simulink library "SUB_ECU_L4_MABX_HW_Interface_PIC_PB"  (R2018a)
settings: Solver=VariableStepAuto  StartTime=0.0  StopTime=10.0  RelTol=1e-3
PostLoadFcn:
  | , if any(exist('dsrtsu_mdlpostloadfcn', 'file') == [2, 3, 6]), try dsrtsu_mdlpostloadfcn('Execute', bdroot); catch fprintf('Error in PostLoadFcn (dsrtsu_mdlpostloadfcn) for model "%s":\n %s\n', bdroot, lasterr); end, end,
undefined symbols (not defined in the file or in its folder): CANR_PROPB_REAX_3_13_CHANNEL_APV, CANR_PROPB_REAX_4_13_CHANNEL_APV, CANR_PROPB_XPR_1_50_CHANNEL_APV, ENUM_CAN_RX_T, ENUM_CAN_TX_T, ENUM_REAX_OPERATION_MODE_T, ENUM_SIGNAL_HEALTH_T, ENUM_XBR_CONTROL_MODE_T, ENUM_XBR_EBI_MODE_T, ENUM_XBR_PASS_THROUGH_ACTIVE_T, ENUM_XBR_PRIORITY_T, ENUM_XPR_INHIBIT_PARK_MANUAL_T, ENUM_XPR_INHIBIT_UNPARK_MANUAL_T, ENUM_XPR_PARK_MANUAL_T, ENUM_XPR_UNPARK_MANUAL_T, PROPB_REAX_1_E4_DES_POS_SIG_SRC_APV, PROPB_REAX_1_E4_DESIRED_OPMODE_APV, PROPB_REAX_1_E4_DESIRED_POSITION_APV, PROPB_REAX_CHANNEL_APV, ptc_matlab_lib
libraries: PTC_MBDS_LIB x293, rtican x158, simulink x61, EmE_MBD_Blockset x38, rti1401lib_dio_type4 x14, simulink_need_slupdate x7, $bdroot x5, rti1401lib_adc_type4 x3, rtmapslib x3, dsa_tcpip_lib x2, SUB_ECU_L4_MABX_HW_Interface_PTC_1571 x1, rtitasklib x1
(part 19 of 49)

== system SUB_ECU_L4_MABX_HW_Interface_PIC_PB/CAN_PIC_PB/CAN_RX_TC1_05/RX_CAN_5 ==
  Enable : Inport
  Bus Creator3 : BusCreator  Inputs=28
  Data Type Conversion10 : DataTypeConversion  OutDataTypeStr=double  SaturateOnIntegerOverflow=on
  Data Type Conversion8 : DataTypeConversion  OutDataTypeStr=boolean  SaturateOnIntegerOverflow=on
  Data Type Conversion9 : DataTypeConversion  OutDataTypeStr=double  SaturateOnIntegerOverflow=on
  TC1_03_05 : rtican/RTICAN Receive (RX)   Reserved1=[]  Reserved2=[]  Reserved3=[]  Reserved4=[]  SfcnMessage=[]  Msg_Struct=[]  BoardTypeNo=[]  BoardNo=[]  ChannelNo=[]  Parameters=[]  DialogFcn=[]  UnitName=[]  Revision=[]  UnitValues=[]  DSProperties=struct('RTI',struct('Version',uint32(5),'BlockType',struct('isSLSource',uint8(1),'isSLSink',uint8(1),'isHWSource',uint8(0),'isHWSink',uint8(0),'isSetup',uint8(0),'isInline',uint8(1),'isNonInline',uint8(0),'isInterrupt',uint8(0),'isChannelwise',uint8(0)),'IOBoardType','RTICAN','UnitType','MESSAGE','Identifier','RX','DialogType','MSVC','BlockSet','RTICAN','SlaveProcessor','CAN'))  RTIBlockInterface=struct('OutputPortsWidth',int32([1 1 1 1 1 1 1 1 1 1 1 1 1 1 1 1 1 1 1 1 1 1 1 1 1 1 1 1]),'OutputPortsActive',ones(1,28),'OutputPortsName',{{'SPN681_TransGearShiftInhibitReq','SPN682_TransTrqConvLockupDisReq','SPN683_DisengageDrivelineReq','SPN4242_TransRevGearShiftInhibRq','SPN684_RequestedPercClutchSlip','SPN525_TransRequestedGear','SPN685_DisengageDiffLockRqFrAx1','SPN686_DisengageDiffLockRqFrAx2','SPN687_DisengageDiffLockRqRrAx1','SPN688_DisengageDiffLockRqRrAx2','SPN689_DisengageDiffLockRqC','SPN690_DisengageDiffLockRqCF','SPN691_DisengageDiffLockRqCR','SPN5762_TransLoadRedInhibitRq','SPN1852_TransmissionMode1','SPN1853_TransmissionMode2','SPN1854_TransmissionMode3','SPN1855_TransmissionMode4','SPN7695_TransAutoNeutralRequest','SPN4255_TransRequestedLaunchGear','SPN2985_TransShiftSelDispModeSw','SPN4246_TransmissionMode5','SPN4247_TransmissionMode6','SPN4248_TransmissionMode7','SPN4249_TransmissionMode8',['RX status'],['RX time'],['RX delta time']}},'OutputPortsDataType',{{'SS_DOUBLE','SS_DOUBLE','SS_DOUBLE','SS_DOUBLE','SS_DOUBLE','SS_DOUBLE','SS_DOUBLE','SS_DOUBLE','SS_DOUBLE','SS_DOUBLE','SS_DOUBLE','SS_DOUBLE','SS_DOUBLE','SS_DOUBLE','SS_DOUBLE','SS_DOUBLE','SS_DOUBLE','SS_DOUBLE','SS_DOUBLE','SS_DOUBLE','SS_DOUBLE','SS_DOUBLE','SS_DOUBLE','SS_DOUBLE','SS_DOUBLE','SS_DOUBLE','SS_DOUBLE','SS_DOUBLE'}},'OutputPortsLabel',{{'SPN681_TransGearShiftInhibitReq','SPN682_TransTrqConvLockupDisReq','SPN683_DisengageDrivelineReq','SPN4242_TransRevGearShiftInhibRq','SPN684_RequestedPercClutchSlip','SPN525_TransRequestedGear','SPN685_DisengageDiffLockRqFrAx1','SPN686_DisengageDiffLockRqFrAx2','SPN687_DisengageDiffLockRqRrAx1','SPN688_DisengageDiffLockRqRrAx2','SPN689_DisengageDiffLockRqC','SPN690_DisengageDiffLockRqCF','SPN691_DisengageDiffLockRqCR','SPN5762_TransLoadRedInhibitRq','SPN1852_TransmissionMode1','SPN1853_TransmissionMode2','SPN1854_TransmissionMode3','SPN1855_TransmissionMode4','SPN7695_TransAutoNeutralRequest','SPN4255_TransRequestedLaunchGear','SPN2985_TransShiftSelDispModeSw','SPN4246_TransmissionMode5','SPN4247_TransmissionMode6','SPN4248_TransmissionMode7','SPN4249_TransmissionMode8','','',''}},'OutputPortsLabelMode','ON','InputPortsWidth',int32(0),'InputPortsActive',0,'DialogFcn','rtican_message_interface_gui','BlockDisplay',{{'','center'}},'IconTransparency','on','ParameterTunableNames',{{}},'InitLevel',3,'BlockName',struct('Token',{{'TC1_03_05'}}),'SampleTime',{{-1}},'TriggerPort',{{'none'}},'EnablePort',{{'yes'}})  RTIBlockParameters="struct('BoardTypeNo',{{1,'OFF',[]}},'BoardNo',{{3,'ON',[1 16]}},'ChannelNo',{{1,'ON',[1 2]}},'Parameters',{{struct('DataFileSupport',struct('DataFileSelectedMaster',1,'DataFileSelectedLocal',0,'DataFileName',['c:\\users\\gavin.coelho\\repos\\l4 svn\\branches\\gennaro\\project_l4\\src\\projectlibrary\\dbc\\mabx_can4_chrisbaltonallstandard.dbc|c:\\users\\gavin.coelho\\repos\\l4 svn\\branches\\gennaro\\project_l4\\src\\projectlibrary\\dbc\\mabx_can4.dbc|'],'DataFileDate',{{{''}}},'SelectedFile',['<no file selected>']),'Options',struct('StatusSelected',1,'TimeSelected',1,'DeltaTimeSelected',1,'BytePortSelected',0,'MessageLengthSelected',0,'TriggerPort',struct('Selected',0,'TriggerType',0),'UserCoding',struct('Selected',0,'InterfaceFile','UserDecodingFile','FcnName','UserDecodeFcn','InportSelected',0,'InportWidth',1,'OutportSelected',0,'OutportWidth',1),'EnablePortSelected',1,'SignalOnPortnameSelected',1,'UseRXService',1),'Message',struct('MsgOnBlocknameSelected',1,'MsgName','TC1_03_05','MsgIdFormat',1,'MsgId',201392901,'MsgLength',8,'NumSignals',25,'SampleTime',-1,'Signal',struct('SgnName',{'SPN681_TransGearShiftInhibitReq','SPN682_TransTrqConvLockupDisReq','SPN683_DisengageDrivelineReq','SPN4242_TransRevGearShiftInhibRq','SPN684_RequestedPercClutchSlip','SPN525_TransRequestedGear','SPN685_DisengageDiffLockRqFrAx1','SPN686_DisengageDiffLockRqFrAx2','SPN687_DisengageDiffLockRqRrAx1','SPN688_DisengageDiffLockRqRrAx2','SPN689_DisengageDiffLockRqC','SPN690_DisengageDiffLockRqCF','SPN691_DisengageDiffLockRqCR','SPN5762_TransLoadRedInhibitRq','SPN1852_TransmissionMode1','SPN1853_TransmissionMode2','SPN1854_TransmissionMode3','SPN1855_TransmissionMode4','SPN7695_TransAutoNeutralRequest','SPN4255_TransRequestedLaunchGear','SPN2985_TransShiftSelDispModeSw','SPN4246_TransmissionMode5','SPN4247_TransmissionMode6','SPN4248_TransmissionMode7','SPN4249_TransmissionMode8'},'SgnStartBit',{0,2,4,6,8,16,24,26,28,30,32,34,36,38,40,42,44,46,48,50,54,56,58,60,62},'SgnLength',{2,2,2,2,8,8,2,2,2,2,2,2,2,2,2,2,2,2,2,4,2,2,2,2,2},'SgnType',{0,0,0,0,0,0,0,0,0,0,0,0,0,0,0,0,0,0,0,0,0,0,0,0,0},'ModeValue',{-1,-1,-1,-1,-1,-1,-1,-1,-1,-1,-1,-1,-1,-1,-1,-1,-1,-1,-1,-1,-1,-1,-1,-1,-1},'DataType',{0,0,0,0,0,0,0,0,0,0,0,0,0,0,0,0,0,0,0,0,0,0,0,0,0},'ByteLayout',{0,0,0,0,0,0,0,0,0,0,0,0,0,0,0,0,0,0,0,0,0,0,0,0,0},'Factor',{1,1,1,1,0.4,1,1,1,1,1,1,1,1,1,1,1,1,1,1,1,1,1,1,1,1},'Offset',{0,0,0,0,0,-125,0,0,0,0,0,0,0,0,0,0,0,0,0,0,0,0,0,0,0},'SgnComment',{{['Command signal to inhibit gear shifts.']},{['Command signal to prevent torque converter lockup, which may cause problems in certain circumstances for ASR.']},{''},{['Allows devices external to the normal transmission shift selector system to request the transmission to inhibit shifts into any Reverse gear and force the transmission into Neutral if it is currently in Reverse or attempting to shift to Reverse.']},{['Parameter which represents the percent clutch slip requested by a device.']},{['Gear requested by the operator, ABS, or engine.']},{['Command signal used to disengage the various differential locks, e.g., to allow an undistributed individual wheel control by ABS.  The differential locks are located as defined in Figure SPN564_A.']},{['Command signal used to disengage the various differential locks, e.g., to allow an undistributed individual wheel control by ABS.  The differential locks are located as defined in Figure SPN564_A']},{['Command signal used to disengage the various differential locks, e.g., to allow an undistributed individual wheel control by ABS.  The differential locks are located as defined in Figure SPN564_A']},{['Command signal used to disengage the various differential locks, e.g., to allow an undistributed individual wheel control by ABS.  The differential locks are located as defined in Figure SPN564_A']},{['Command signal used to disengage the various differential locks, e.g., to allow an undistributed individual wheel control by ABS.  The differential locks are located as defined in Figure SPN564_A']},{['Command signal used to disengage the various differential locks, e.g., to allow an undistributed individual wheel control by ABS.  The differential locks are located as defined in Figure SPN564_A.']},{['Command signal used to disengage the various differential locks, e.g., to allow an undistributed individual wheel control by ABS.  The differential locks are located as defined in Figure SPN564_A.']},{['Request signal to the transmission to inhibit activation of load reduction functions.']},{['Indicates whether transmission mode 1 is enabled.  Modes are manufacturer specific and are not necessarily mutually exclusive.  See also SPN 2536.']},{['Indicates whether transmission mode 2 is enabled.  Modes are manufacturer specific and are not necessarily mutually exclusive.  See also SPN 2537.']},{['Indicates whether transmission mode 3 is enabled.  Modes are manufacturer specific and are not necessarily mutually exclusive.  See also SPN 2538.']},{['Indicates whether transmission mode 4 is enabled.  Modes are manufacturer specific and are not necessarily mutually exclusive.  See also SPN 2539.']},{['This parameter conveys a vehicle system desire to override the operator’s current shift selector request (e.g. Drive, Reverse) and shift the transmission into Neutral']},{['Initial gear for the transmission to start out in when the vehicle is launched from a standing stop, as specified by the vehicle operator or vehicle system.']},{['Status of the operator’s switch used to ‘toggle’ through multiple display modes of a shift selector display.']},{['Indicates whether transmission mode 5 is enabled. Modes are manufacturer specific and are not necessarily mutually exclusive. See also SPN 4250.']},{['Indicates whether transmission mode 6 is enabled. Modes are manufacturer specific and are not necessarily mutually exclusive. See also SPN 4251.']},{['Indicates whether transmission mode 7 is enabled. Modes are manufacturer specific and are not necessarily mutually exclusive. See also SPN 4252.']},{['Indicates whether transmission mode 8 is enabled. Modes are manufacturer specific and are not necessarily mutually exclusive. See also SPN 4253.']}},'SgnUnit',{'','','','','%','','','','','','','','','','','','','','','','','','','',''},'Min',{0,0,0,0,0,0,0,0,0,0,0,0,0,0,0,0,0,0,0,0,0,0,0,0,0},'Max',{0,0,0,0,0,0,0,0,0,0,0,0,0,0,0,0,0,0,0,0,0,0,0,0,0},'SLDataType',{'SS_DOUBLE','SS_DOUBLE','SS_DOUBLE','SS_DOUBLE','SS_DOUBLE','SS_DOUBLE','SS_DOUBLE','SS_DOUBLE','SS_DOUBLE','SS_DOUBLE','SS_DOUBLE','SS_DOUBLE','SS_DOUBLE','SS_DOUBLE','SS_DOUBLE','SS_DOUBLE','SS_DOUBLE','SS_DOUBLE','SS_DOUBLE','SS_DOUBLE','SS_DOUBLE','SS_DOUBLE','SS_DOUBLE','SS_DOUBLE','SS_DOUBLE'}),'MsgIdNumFormat',1,'MsgComment',{{['Transmission Control 1']}}),'Version',1.2,'general',struct('isFromLib',0)),'OFF',[]}},'GroupId',{{struct('Group',{{'RTICAN'}},'No',5,'Behavior',{{'NAMECHANGE'}},'BlockType',{{'SINK'}},'NameChangeFlag',0),'OFF',[]}},'SFcnRTICANMessage',{{struct('MsgType','RX','SFcnPortType','Scalar','MsgName','TC1_03_05','MsgIdFormat','XTD','MsgId',201392901,'MsgLength',8,'NumSignals',25,'SampleTime',-1,'Signal',struct('SgnName',{'SPN681_TransGearShiftInhibitReq','SPN682_TransTrqConvLockupDisReq','SPN683_DisengageDrivelineReq','SPN4242_TransRevGearShiftInhibRq','SPN684_RequestedPercClutchSlip','SPN525_TransRequestedGear','SPN685_DisengageDiffLockRqFrAx1','SPN686_DisengageDiffLockRqFrAx2','SPN687_DisengageDiffLockRqRrAx1','SPN688_DisengageDiffLockRqRrAx2','SPN689_DisengageDiffLockRqC','SPN690_DisengageDiffLockRqCF','SPN691_DisengageDiffLockRqCR','SPN5762_TransLoadRedInhibitRq','SPN1852_TransmissionMode1','SPN1853_TransmissionMode2','SPN1854_TransmissionMode3','SPN1855_TransmissionMode4','SPN7695_TransAutoNeutralRequest','SPN4255_TransRequestedLaunchGear','SPN2985_TransShiftSelDispModeSw','SPN4246_TransmissionMode5','SPN4247_TransmissionMode6','SPN4248_TransmissionMode7','SPN4249_TransmissionMode8'},'SgnStartBit',{0,2,4,6,8,16,24,26,28,30,32,34,36,38,40,42,44,46,48,50,54,56,58,60,62},'SgnLength',{2,2,2,2,8,8,2,2,2,2,2,2,2,2,2,2,2,2,2,4,2,2,2,2,2},'SgnType',{'standard','standard','standard','standard','standard','standard','standard','standard','standard','standard','standard','standard','standard','standard','standard','standard','standard','standard','standard','standard','standard','standard','standard','standard','standard'},'ModeValue',{-1,-1,-1,-1,-1,-1,-1,-1,-1,-1,-1,-1,-1,-1,-1,-1,-1,-1,-1,-1,-1,-1,-1,-1,-1},'DataType',{['unsigned int'],['unsigned int'],['unsigned int'],['unsigned int'],['unsigned int'],['unsigned int'],['unsigned int'],['unsigned int'],['unsigned int'],['unsigned int'],['unsigned int'],['unsigned int'],['unsigned int'],['unsigned int'],['unsigned int'],['unsigned int'],['unsigned int'],['unsigned int'],['unsigned int'],['unsigned int'],['unsigned int'],['unsigned int'],['unsigned int'],['unsigned int'],['unsigned int']},'ByteLayout',{['little endian'],['little endian'],['little endian'],['little endian'],['little endian'],['little endian'],['little endian'],['little endian'],['little endian'],['little endian'],['little endian'],['little endian'],['little endian'],['little endian'],['little endian'],['little endian'],['little endian'],['little endian'],['little endian'],['little endian'],['little endian'],['little endian'],['little endian'],['little endian'],['little endian']},'Factor',{1,1,1,1,0.4,1,1,1,1,1,1,1,1,1,1,1,1,1,1,1,1,1,1,1,1},'Offset',{0,0,0,0,0,-125,0,0,0,0,0,0,0,0,0,0,0,0,0,0,0,0,0,0,0},'SLDataType',{'SS_DOUBLE','SS_DOUBLE','SS_DOUBLE','SS_DOUBLE','SS_DOUBLE','SS_DOUBLE','SS_DOUBLE','SS_DOUBLE','SS_DOUBLE','SS_DOUBLE','SS_DOUBLE','SS_DOUBLE','SS_DOUBLE','SS_DOUBLE','SS_DOUBLE','SS_DOUBLE','SS_DOUBLE','SS_DOUBLE','SS_DOUBLE','SS_DOUBLE','SS_DOUBLE','SS_DOUBLE','SS_DOUBLE','SS_DOUBLE','SS_DOUBLE'}),'StatusSelected','yes','TimeSelected','yes','DeltaTimeSelected','yes','BytePortSelected','no','MessageLengthSelected','no','TriggerPort',struct('Selected','no','TriggerType',0),'UserCoding',struct('Selected','no','InterfaceFile','UserDecodingFile','FcnName','UserDecodeFcn','InportSelected','no','InportWidth',1,'OutportSelected','no','OutportWidth',1),'EnablePortSelected','yes','UseRXService','yes','BoardType','DS1','BoardNo',3,'ControllerNo',1),'OFF',[]}},'TLCFileName',{{'rtican_rx_message','OFF',[]}})"  RTISFcnParameters=struct('SFcnRTICANMessage','struct','TLCFileName','char')  RTIBlockParaDefault=struct('BoardTypeNo',4302,'BoardNo',1,'ChannelNo',1,'Parameters',struct('DataFileSupport',struct('DataFileSelectedMaster',0,'DataFileSelectedLocal',0,'DataFileName','','DataFileDate','','SelectedFile',['<no file selected>']),'Options',struct('StatusSelected',1,'TimeSelected',1,'DeltaTimeSelected',1,'BytePortSelected',0,'MessageLengthSelected',0,'TriggerPort',struct('Selected',0,'TriggerType','rising'),'UserCoding',struct('Selected',0,'InterfaceFile','UserDecodingFile','FcnName','UserDecodeFcn','InportSelected',0,'InportWidth',1,'OutportSelected',0,'OutportWidth',1),'EnablePortSelected',0,'SignalOnPortnameSelected',1,'UseRXService',0),'Message',struct('MsgOnBlocknameSelected',0,'MsgName',['RX Message'],'MsgIdFormat',0,'MsgId',100,'MsgLength',8,'NumSignals',1,'SampleTime',-1,'Signal',struct('SgnName',['RX signal'],'SgnStartBit',0,'SgnLength',8,'SgnType',0,'ModeValue',-1,'DataType',0,'SLDataType','SS_DOUBLE','ByteLayout',0,'Factor',1,'Offset',0,'Min',0,'Max',255,'SgnComment',{{}},'SgnUnit',''),'MsgIdNumFormat',0,'MsgComment',{{''}}),'Version',1.2,'general',struct('isFromLib',1)),'GroupId',struct('Group',{{'RTICAN'}},'No',1,'Behavior',{{'NAMECHANGE'}},'BlockType',{{'SINK'}},'NameChangeFlag',0),'SFcnRTICANMessage',struct('MsgType','RX','MsgName',['RX Message'],'MsgIdFormat','STD','MsgId',100,'MsgLength',8,'NumSignals',1,'SampleTime',-1,'Signal',struct('SgnName',['RX signal'],'SgnStartBit',0,'SgnLength',8,'SgnType','standard','ModeValue',-1,'DataType',['unsigned int'],'ByteLayout',['little endian'],'SLDataType','SS_DOUBLE','Factor',1,'Offset',0),'StatusSelected','yes','TimeSelected','yes','DeltaTimeSelected','yes','BytePortSelected','no','MessageLengthSelected','no','EnablePortSelected','no','UserCoding',struct('Selected','no','InterfaceFile','UserDecodingFile','FcnName','UserDecodeFcn','InportSelected','no','InportWidth',1,'OutportSelected','no','OutportWidth',1),'TriggerPort',struct('Selected','no','TriggerType','rising'),'UseRXService','no','BoardType','DS4302','BoardNo',1,'ControllerNo',1,'SFcnPortType','Scalar'),'TLCFileName','rtican_rx_message')
      settings: AttributesFormatString=Group Id: RTICAN5\n  SourceProductName=dSPACE RTI CAN Blockset
  TC1_05 : Outport
  wires:
  Data Type Conversion9/1 -> Bus Creator3/27  "RX_time"
  Data Type Conversion10/1 -> Bus Creator3/28  "RX_delta_time"
  Data Type Conversion8/1 -> Bus Creator3/26  "RX_status"
  TC1_03_05/26 -> Data Type Conversion8/1
  TC1_03_05/27 -> Data Type Conversion9/1
  TC1_03_05/28 -> Data Type Conversion10/1
  Enable/1 -> TC1_03_05/Enable
  Bus Creator3/1 -> TC1_05/1  "TC1_05"
  TC1_03_05/23 -> Bus Creator3/23  "SPN4247_TransmissionMode6"
  TC1_03_05/24 -> Bus Creator3/24  "SPN4248_TransmissionMode7"
  TC1_03_05/25 -> Bus Creator3/25  "SPN4249_TransmissionMode8"
  TC1_03_05/22 -> Bus Creator3/22  "SPN4246_TransmissionMode5"
  TC1_03_05/21 -> Bus Creator3/21  "SPN2985_TransShiftSelDispModeSw"
  TC1_03_05/7 -> Bus Creator3/7  "SPN685_DisengageDiffLockRqFrAx1"
  TC1_03_05/18 -> Bus Creator3/18  "SPN1855_TransmissionMode4"
  TC1_03_05/19 -> Bus Creator3/19  "SPN7695_TransAutoNeutralRequest"
  TC1_03_05/8 -> Bus Creator3/8  "SPN686_DisengageDiffLockRqFrAx2"
  TC1_03_05/12 -> Bus Creator3/12  "SPN690_DisengageDiffLockRqCF"
  TC1_03_05/16 -> Bus Creator3/16  "SPN1853_TransmissionMode2"
  TC1_03_05/9 -> Bus Creator3/9  "SPN687_DisengageDiffLockRqRrAx1"
  TC1_03_05/10 -> Bus Creator3/10  "SPN688_DisengageDiffLockRqRrAx2"
  TC1_03_05/11 -> Bus Creator3/11  "SPN689_DisengageDiffLockRqC"
  TC1_03_05/13 -> Bus Creator3/13  "SPN691_DisengageDiffLockRqCR"
  TC1_03_05/20 -> Bus Creator3/20  "SPN4255_TransRequestedLaunchGear"
  TC1_03_05/15 -> Bus Creator3/15  "SPN1852_TransmissionMode1"
  TC1_03_05/17 -> Bus Creator3/17  "SPN1854_TransmissionMode3"
  TC1_03_05/14 -> Bus Creator3/14  "SPN5762_TransLoadRedInhibitRq"
  TC1_03_05/3 -> Bus Creator3/3  "SPN683_DisengageDrivelineReq"
  TC1_03_05/6 -> Bus Creator3/6  "SPN525_TransRequestedGear"
  TC1_03_05/4 -> Bus Creator3/4  "SPN4242_TransRevGearShiftInhibRq"
  TC1_03_05/5 -> Bus Creator3/5  "SPN684_RequestedPercClutchSlip"
  TC1_03_05/1 -> Bus Creator3/1  "SPN681_TransGearShiftInhibitReq"
  TC1_03_05/2 -> Bus Creator3/2  "SPN682_TransTrqConvLockupDisReq"

== system SUB_ECU_L4_MABX_HW_Interface_PIC_PB/CAN_PIC_PB/CAN_RX_VDC1_0B/RX_CAN_1 ==
  Enable : Inport
  Bus Creator3 : BusCreator  Inputs=10
  Data Type Conversion10 : DataTypeConversion  OutDataTypeStr=double  SaturateOnIntegerOverflow=on
  Data Type Conversion8 : DataTypeConversion  OutDataTypeStr=boolean  SaturateOnIntegerOverflow=on
  Data Type Conversion9 : DataTypeConversion  OutDataTypeStr=double  SaturateOnIntegerOverflow=on
  VDC1_0B_ : rtican/RTICAN Receive (RX)   Reserved1=[]  Reserved2=[]  Reserved3=[]  Reserved4=[]  SfcnMessage=[]  Msg_Struct=[]  BoardTypeNo=[]  BoardNo=[]  ChannelNo=[]  Parameters=[]  DialogFcn=[]  UnitName=[]  Revision=[]  UnitValues=[]  DSProperties=struct('RTI',struct('Version',uint32(5),'BlockType',struct('isSLSource',uint8(1),'isSLSink',uint8(1),'isHWSource',uint8(0),'isHWSink',uint8(0),'isSetup',uint8(0),'isInline',uint8(1),'isNonInline',uint8(0),'isInterrupt',uint8(0),'isChannelwise',uint8(0)),'IOBoardType','RTICAN','UnitType','MESSAGE','Identifier','RX','DialogType','MSVC','BlockSet','RTICAN','SlaveProcessor','CAN'))  RTIBlockInterface=struct('OutputPortsWidth',int32([1 1 1 1 1 1 1 1 1 1]),'OutputPortsActive',[1 1 1 1 1 1 1 1 1 1],'OutputPortsName',{{'VDCInformationSignal','VDCFullyOperational','VDCBrakeLightRq','ROPEngCtrlActive','ROPBrakeCtrlActive','YCEngCtrlActive','YCBrakeCtrlActive',['RX status'],['RX time'],['RX delta time']}},'OutputPortsDataType',{{'SS_DOUBLE','SS_DOUBLE','SS_DOUBLE','SS_DOUBLE','SS_DOUBLE','SS_DOUBLE','SS_DOUBLE','SS_DOUBLE','SS_DOUBLE','SS_DOUBLE'}},'OutputPortsLabel',{{'VDCInformationSignal','VDCFullyOperational','VDCBrakeLightRq','ROPEngCtrlActive','ROPBrakeCtrlActive','YCEngCtrlActive','YCBrakeCtrlActive','','',''}},'OutputPortsLabelMode','ON','InputPortsWidth',int32(0),'InputPortsActive',0,'DialogFcn','rtican_message_interface_gui','BlockDisplay',{{'','center'}},'IconTransparency','on','ParameterTunableNames',{{}},'InitLevel',3,'BlockName',struct('Token',{{'VDC1_0B'}}),'SampleTime',{{-1}},'TriggerPort',{{'none'}},'EnablePort',{{'yes'}})  RTIBlockParameters=struct('BoardTypeNo',{{1,'OFF',[]}},'BoardNo',{{1,'ON',[1 16]}},'ChannelNo',{{1,'ON',[1 2]}},'Parameters',{{struct('DataFileSupport',struct('DataFileSelectedMaster',1,'DataFileSelectedLocal',0,'DataFileName',['c:\users\gavin.coelho\repos\l4 svn\branches\gennaro\project_l4\src\projectlibrary\dbc\mabx_can1.dbc|c:\users\gavin.coelho\repos\l4 svn\branches\gennaro\project_l4\src\projectlibrary\dbc\j1939_famosdbcwithfusion.dbc|'],'DataFileDate',{{{['31-Jan-2018 07:14:07']},{['31-Jan-2018 07:14:07']}}},'SelectedFile','dbc\j1939_famosdbcwithfusion.dbc','InterfaceFcn','rtican_dbc_file_parser'),'Options',struct('StatusSelected',1,'TimeSelected',1,'DeltaTimeSelected',1,'BytePortSelected',0,'MessageLengthSelected',0,'TriggerPort',struct('Selected',0,'TriggerType',0),'UserCoding',struct('Selected',0,'InterfaceFile','UserDecodingFile','FcnName','UserDecodeFcn','InportSelected',0,'InportWidth',1,'OutportSelected',0,'OutportWidth',1),'EnablePortSelected',1,'SignalOnPortnameSelected',1,'UseRXService',1),'Message',struct('MsgOnBlocknameSelected',1,'MsgName','VDC1_0B','MsgIdFormat',1,'MsgId',419319563,'MsgLength',8,'NumSignals',7,'SampleTime',-1,'Signal',struct('SgnName',{'VDCInformationSignal','VDCFullyOperational','VDCBrakeLightRq','ROPEngCtrlActive','ROPBrakeCtrlActive','YCEngCtrlActive','YCBrakeCtrlActive'},'SgnStartBit',{0,2,4,8,10,12,14},'SgnLength',{2,2,2,2,2,2,2},'SgnType',{0,0,0,0,0,0,0},'ModeValue',{-1,-1,-1,-1,-1,-1,-1},'DataType',{0,0,0,0,0,0,0},'ByteLayout',{0,0,0,0,0,0,0},'Factor',{1,1,1,1,1,1,1},'Offset',{0,0,0,0,0,0,0},'SgnComment',{{['This parameter commands the VDC information signal, for example a dash lamp.']},{['Signal that indicates whether VDC is fully operational or whether its functionality is reduced by a permanent or temporary']},{['Indicates whether VDC requests to turn the vehicle brake lights on']},{['State Signal which indicates that the Roll Over Prevention (ROP) has commanded engine control to be active.']},{['State signal which indicates that Roll over Prevention (ROP) has activated brake control.']},{['State Signal which indicates that the Yaw Control (YC) has commanded engine control to be active.']},{['State signal which indicates that Yaw Control (YC) has activated brake control.']}},'SgnUnit',{'','','','','','',''},'Min',{0,0,0,0,0,0,0},'Max',{3,3,3,3,3,3,3},'SLDataType',{'SS_DOUBLE','SS_DOUBLE','SS_DOUBLE','SS_DOUBLE','SS_DOUBLE','SS_DOUBLE','SS_DOUBLE'}),'MsgIdNumFormat',1,'MsgComment',{{['Vehicle Dynamic Stability Control 1']}}),'Version',1.2,'general',struct('isFromLib',0)),'OFF',[]}},'GroupId',{{struct('Group',{{'RTICAN'}},'No',1,'Behavior',{{'NAMECHANGE'}},'BlockType',{{'SINK'}},'NameChangeFlag',0),'OFF',[]}},'SFcnRTICANMessage',{{struct('MsgType','RX','SFcnPortType','Scalar','MsgName','VDC1_0B','MsgIdFormat','XTD','MsgId',419319563,'MsgLength',8,'NumSignals',7,'SampleTime',-1,'Signal',struct('SgnName',{'VDCInformationSignal','VDCFullyOperational','VDCBrakeLightRq','ROPEngCtrlActive','ROPBrakeCtrlActive','YCEngCtrlActive','YCBrakeCtrlActive'},'SgnStartBit',{0,2,4,8,10,12,14},'SgnLength',{2,2,2,2,2,2,2},'SgnType',{'standard','standard','standard','standard','standard','standard','standard'},'ModeValue',{-1,-1,-1,-1,-1,-1,-1},'DataType',{['unsigned int'],['unsigned int'],['unsigned int'],['unsigned int'],['unsigned int'],['unsigned int'],['unsigned int']},'ByteLayout',{['little endian'],['little endian'],['little endian'],['little endian'],['little endian'],['little endian'],['little endian']},'Factor',{1,1,1,1,1,1,1},'Offset',{0,0,0,0,0,0,0},'SLDataType',{'SS_DOUBLE','SS_DOUBLE','SS_DOUBLE','SS_DOUBLE','SS_DOUBLE','SS_DOUBLE','SS_DOUBLE'}),'StatusSelected','yes','TimeSelected','yes','DeltaTimeSelected','yes','BytePortSelected','no','MessageLengthSelected','no','TriggerPort',struct('Selected','no','TriggerType',0),'UserCoding',struct('Selected','no','InterfaceFile','UserDecodingFile','FcnName','UserDecodeFcn','InportSelected','no','InportWidth',1,'OutportSelected','no','OutportWidth',1),'EnablePortSelected','yes','UseRXService','yes','BoardType','DS1','BoardNo',1,'ControllerNo',1),'OFF',[]}},'TLCFileName',{{'rtican_rx_message','OFF',[]}})  RTISFcnParameters=struct('SFcnRTICANMessage','struct','TLCFileName','char')  RTIBlockParaDefault=struct('BoardTypeNo',4302,'BoardNo',1,'ChannelNo',1,'Parameters',struct('DataFileSupport',struct('DataFileSelectedMaster',0,'DataFileSelectedLocal',0,'DataFileName','','DataFileDate','','SelectedFile',['<no file selected>']),'Options',struct('StatusSelected',1,'TimeSelected',1,'DeltaTimeSelected',1,'BytePortSelected',0,'MessageLengthSelected',0,'TriggerPort',struct('Selected',0,'TriggerType','rising'),'UserCoding',struct('Selected',0,'InterfaceFile','UserDecodingFile','FcnName','UserDecodeFcn','InportSelected',0,'InportWidth',1,'OutportSelected',0,'OutportWidth',1),'EnablePortSelected',0,'SignalOnPortnameSelected',1,'UseRXService',0),'Message',struct('MsgOnBlocknameSelected',0,'MsgName',['RX Message'],'MsgIdFormat',0,'MsgId',100,'MsgLength',8,'NumSignals',1,'SampleTime',-1,'Signal',struct('SgnName',['RX signal'],'SgnStartBit',0,'SgnLength',8,'SgnType',0,'ModeValue',-1,'DataType',0,'SLDataType','SS_DOUBLE','ByteLayout',0,'Factor',1,'Offset',0,'Min',0,'Max',255,'SgnComment',{{}},'SgnUnit',''),'MsgIdNumFormat',0,'MsgComment',{{''}}),'Version',1.2,'general',struct('isFromLib',1)),'GroupId',struct('Group',{{'RTICAN'}},'No',1,'Behavior',{{'NAMECHANGE'}},'BlockType',{{'SINK'}},'NameChangeFlag',0),'SFcnRTICANMessage',struct('MsgType','RX','MsgName',['RX Message'],'MsgIdFormat','STD','MsgId',100,'MsgLength',8,'NumSignals',1,'SampleTime',-1,'Signal',struct('SgnName',['RX signal'],'SgnStartBit',0,'SgnLength',8,'SgnType','standard','ModeValue',-1,'DataType',['unsigned int'],'ByteLayout',['little endian'],'SLDataType','SS_DOUBLE','Factor',1,'Offset',0),'StatusSelected','yes','TimeSelected','yes','DeltaTimeSelected','yes','BytePortSelected','no','MessageLengthSelected','no','EnablePortSelected','no','UserCoding',struct('Selected','no','InterfaceFile','UserDecodingFile','FcnName','UserDecodeFcn','InportSelected','no','InportWidth',1,'OutportSelected','no','OutportWidth',1),'TriggerPort',struct('Selected','no','TriggerType','rising'),'UseRXService','no','BoardType','DS4302','BoardNo',1,'ControllerNo',1,'SFcnPortType','Scalar'),'TLCFileName','rtican_rx_message')
      settings: AttributesFormatString=Group Id: RTICAN1\n  SourceProductName=dSPACE RTI CAN Blockset
  VDC1_0B : Outport
  wires:
  Data Type Conversion9/1 -> Bus Creator3/9  "RX_time"
  Data Type Conversion10/1 -> Bus Creator3/10  "RX_delta_time"
  Data Type Conversion8/1 -> Bus Creator3/8  "RX_status"
  VDC1_0B_/8 -> Data Type Conversion8/1
  VDC1_0B_/9 -> Data Type Conversion9/1
  VDC1_0B_/10 -> Data Type Conversion10/1
  Enable/1 -> VDC1_0B_/Enable
  Bus Creator3/1 -> VDC1_0B/1  "VDC1_0B"
  VDC1_0B_/1 -> Bus Creator3/1  "VDCInformationSignal"
  VDC1_0B_/2 -> Bus Creator3/2  "VDCFullyOperational"
  VDC1_0B_/3 -> Bus Creator3/3  "VDCBrakeLightRq"
  VDC1_0B_/4 -> Bus Creator3/4  "ROPEngCtrlActive"
  VDC1_0B_/5 -> Bus Creator3/5  "ROPBrakeCtrlActive"
  VDC1_0B_/6 -> Bus Creator3/6  "YCEngCtrlActive"
  VDC1_0B_/7 -> Bus Creator3/7  "YCBrakeCtrlActive"

== system SUB_ECU_L4_MABX_HW_Interface_PIC_PB/CAN_PIC_PB/CAN_RX_VDC2_0B/RX_CAN_1 ==
  Enable : Inport
  Bus Creator3 : BusCreator  Inputs=9
  Data Type Conversion10 : DataTypeConversion  OutDataTypeStr=double  SaturateOnIntegerOverflow=on
  Data Type Conversion8 : DataTypeConversion  OutDataTypeStr=boolean  SaturateOnIntegerOverflow=on
  Data Type Conversion9 : DataTypeConversion  OutDataTypeStr=double  SaturateOnIntegerOverflow=on
  VDC2_0B1 : rtican/RTICAN Receive (RX)   Reserved1=[]  Reserved2=[]  Reserved3=[]  Reserved4=[]  SfcnMessage=[]  Msg_Struct=[]  BoardTypeNo=[]  BoardNo=[]  ChannelNo=[]  Parameters=[]  DialogFcn=[]  UnitName=[]  Revision=[]  UnitValues=[]  DSProperties=struct('RTI',struct('Version',uint32(5),'BlockType',struct('isSLSource',uint8(1),'isSLSink',uint8(1),'isHWSource',uint8(0),'isHWSink',uint8(0),'isSetup',uint8(0),'isInline',uint8(1),'isNonInline',uint8(0),'isInterrupt',uint8(0),'isChannelwise',uint8(0)),'IOBoardType','RTICAN','UnitType','MESSAGE','Identifier','RX','DialogType','MSVC','BlockSet','RTICAN','SlaveProcessor','CAN'))  RTIBlockInterface=struct('OutputPortsWidth',int32([1 1 1 1 1 1 1 1 1]),'OutputPortsActive',[1 1 1 1 1 1 1 1 1],'OutputPortsName',{{'SteerWheelAngle','SteerWheelTurnCounter','SteerWheelAngleSensorType','YawRate','LateralAcceleration','LongitudinalAcceleration',['RX status'],['RX time'],['RX delta time']}},'OutputPortsDataType',{{'SS_DOUBLE','SS_DOUBLE','SS_DOUBLE','SS_DOUBLE','SS_DOUBLE','SS_DOUBLE','SS_DOUBLE','SS_DOUBLE','SS_DOUBLE'}},'OutputPortsLabel',{{'SteerWheelAngle','SteerWheelTurnCounter','SteerWheelAngleSensorType','YawRate','LateralAcceleration','LongitudinalAcceleration','','',''}},'OutputPortsLabelMode','ON','InputPortsWidth',int32(0),'InputPortsActive',0,'DialogFcn','rtican_message_interface_gui','BlockDisplay',{{'','center'}},'IconTransparency','on','ParameterTunableNames',{{}},'InitLevel',3,'BlockName',struct('Token',{{'VDC2_0B'}}),'SampleTime',{{-1}},'TriggerPort',{{'none'}},'EnablePort',{{'yes'}})  RTIBlockParameters=struct('BoardTypeNo',{{1,'OFF',[]}},'BoardNo',{{1,'ON',[1 16]}},'ChannelNo',{{1,'ON',[1 2]}},'Parameters',{{struct('DataFileSupport',struct('DataFileSelectedMaster',1,'DataFileSelectedLocal',0,'DataFileName',['c:\users\gavin.coelho\repos\l4 svn\branches\gennaro\project_l4\src\projectlibrary\dbc\mabx_can1.dbc|c:\users\gavin.coelho\repos\l4 svn\branches\gennaro\project_l4\src\projectlibrary\dbc\j1939_famosdbcwithfusion.dbc|'],'DataFileDate',['03-Apr-2017 12:55:40'],'SelectedFile',['<no file selected>'],'InterfaceFcn','rtican_dbc_file_parser'),'Options',struct('StatusSelected',1,'TimeSelected',1,'DeltaTimeSelected',1,'BytePortSelected',0,'MessageLengthSelected',0,'TriggerPort',struct('Selected',0,'TriggerType',0),'UserCoding',struct('Selected',0,'InterfaceFile','UserDecodingFile','FcnName','UserDecodeFcn','InportSelected',0,'InportWidth',1,'OutportSelected',0,'OutportWidth',1),'EnablePortSelected',1,'SignalOnPortnameSelected',1,'UseRXService',1),'Message',struct('MsgOnBlocknameSelected',1,'MsgName','VDC2_0B','MsgIdFormat',1,'MsgId',418384139,'MsgLength',8,'NumSignals',6,'SampleTime',-1,'Signal',struct('SgnName',{'SteerWheelAngle','SteerWheelTurnCounter','SteerWheelAngleSensorType','YawRate','LateralAcceleration','LongitudinalAcceleration'},'SgnStartBit',{0,16,22,24,40,56},'SgnLength',{16,6,2,16,16,8},'SgnType',{0,0,0,0,0,0},'ModeValue',{-1,-1,-1,-1,-1,-1},'DataType',{0,0,0,0,0,0},'ByteLayout',{0,0,0,0,0,0},'Factor',{2^-10,1,1,2^-13,2^-11,0.1},'Offset',{-31.374,-32,0,-3.92,-15.687,-12.5},'SgnComment',{{['The main operator`s steering wheel angle (on the steering column, not the actual wheel angle).']},{['Indicates number of steering wheel turns, absolute position or relative position at ignition on.']},{['Indicates whether the steering wheel angle sensor is capable of absolute measuring of the number of steering wheel']},{['Indicates the rotation about the vertical axis.']},{['Indicates a lateral acceleration of the vehicle.']},{['Indicates the longitudinal acceleration of the vehicle.']}},'SgnUnit',{'rad','turns','','rad/s','m/s²','m/s²'},'Min',{-31.374,-32,0,-3.92,-15.687,-12.5},'Max',{31.374,29,3,3.92,15.687,12.5},'SLDataType',{'SS_DOUBLE','SS_DOUBLE','SS_DOUBLE','SS_DOUBLE','SS_DOUBLE','SS_DOUBLE'}),'MsgIdNumFormat',1,'MsgComment',{{['Vehicle Dynamic Stability Control 2']}}),'Version',1.2,'general',struct('isFromLib',0)),'OFF',[]}},'GroupId',{{struct('Group',{{'RTICAN'}},'No',1,'Behavior',{{'NAMECHANGE'}},'BlockType',{{'SINK'}},'NameChangeFlag',0),'OFF',[]}},'SFcnRTICANMessage',{{struct('MsgType','RX','SFcnPortType','Scalar','MsgName','VDC2_0B','MsgIdFormat','XTD','MsgId',418384139,'MsgLength',8,'NumSignals',6,'SampleTime',-1,'Signal',struct('SgnName',{'SteerWheelAngle','SteerWheelTurnCounter','SteerWheelAngleSensorType','YawRate','LateralAcceleration','LongitudinalAcceleration'},'SgnStartBit',{0,16,22,24,40,56},'SgnLength',{16,6,2,16,16,8},'SgnType',{'standard','standard','standard','standard','standard','standard'},'ModeValue',{-1,-1,-1,-1,-1,-1},'DataType',{['unsigned int'],['unsigned int'],['unsigned int'],['unsigned int'],['unsigned int'],['unsigned int']},'ByteLayout',{['little endian'],['little endian'],['little endian'],['little endian'],['little endian'],['little endian']},'Factor',{2^-10,1,1,2^-13,2^-11,0.1},'Offset',{-31.374,-32,0,-3.92,-15.687,-12.5},'SLDataType',{'SS_DOUBLE','SS_DOUBLE','SS_DOUBLE','SS_DOUBLE','SS_DOUBLE','SS_DOUBLE'}),'StatusSelected','yes','TimeSelected','yes','DeltaTimeSelected','yes','BytePortSelected','no','MessageLengthSelected','no','TriggerPort',struct('Selected','no','TriggerType',0),'UserCoding',struct('Selected','no','InterfaceFile','UserDecodingFile','FcnName','UserDecodeFcn','InportSelected','no','InportWidth',1,'OutportSelected','no','OutportWidth',1),'EnablePortSelected','yes','UseRXService','yes','BoardType','DS1','BoardNo',1,'ControllerNo',1),'OFF',[]}},'TLCFileName',{{'rtican_rx_message','OFF',[]}})  RTISFcnParameters=struct('SFcnRTICANMessage','struct','TLCFileName','char')  RTIBlockParaDefault=struct('BoardTypeNo',4302,'BoardNo',1,'ChannelNo',1,'Parameters',struct('DataFileSupport',struct('DataFileSelectedMaster',0,'DataFileSelectedLocal',0,'DataFileName','','DataFileDate','','SelectedFile',['<no file selected>']),'Options',struct('StatusSelected',1,'TimeSelected',1,'DeltaTimeSelected',1,'BytePortSelected',0,'MessageLengthSelected',0,'TriggerPort',struct('Selected',0,'TriggerType','rising'),'UserCoding',struct('Selected',0,'InterfaceFile','UserDecodingFile','FcnName','UserDecodeFcn','InportSelected',0,'InportWidth',1,'OutportSelected',0,'OutportWidth',1),'EnablePortSelected',0,'SignalOnPortnameSelected',1,'UseRXService',0),'Message',struct('MsgOnBlocknameSelected',0,'MsgName',['RX Message'],'MsgIdFormat',0,'MsgId',100,'MsgLength',8,'NumSignals',1,'SampleTime',-1,'Signal',struct('SgnName',['RX signal'],'SgnStartBit',0,'SgnLength',8,'SgnType',0,'ModeValue',-1,'DataType',0,'SLDataType','SS_DOUBLE','ByteLayout',0,'Factor',1,'Offset',0,'Min',0,'Max',255,'SgnComment',{{}},'SgnUnit',''),'MsgIdNumFormat',0,'MsgComment',{{''}}),'Version',1.2,'general',struct('isFromLib',1)),'GroupId',struct('Group',{{'RTICAN'}},'No',1,'Behavior',{{'NAMECHANGE'}},'BlockType',{{'SINK'}},'NameChangeFlag',0),'SFcnRTICANMessage',struct('MsgType','RX','MsgName',['RX Message'],'MsgIdFormat','STD','MsgId',100,'MsgLength',8,'NumSignals',1,'SampleTime',-1,'Signal',struct('SgnName',['RX signal'],'SgnStartBit',0,'SgnLength',8,'SgnType','standard','ModeValue',-1,'DataType',['unsigned int'],'ByteLayout',['little endian'],'SLDataType','SS_DOUBLE','Factor',1,'Offset',0),'StatusSelected','yes','TimeSelected','yes','DeltaTimeSelected','yes','BytePortSelected','no','MessageLengthSelected','no','EnablePortSelected','no','UserCoding',struct('Selected','no','InterfaceFile','UserDecodingFile','FcnName','UserDecodeFcn','InportSelected','no','InportWidth',1,'OutportSelected','no','OutportWidth',1),'TriggerPort',struct('Selected','no','TriggerType','rising'),'UseRXService','no','BoardType','DS4302','BoardNo',1,'ControllerNo',1,'SFcnPortType','Scalar'),'TLCFileName','rtican_rx_message')
      settings: AttributesFormatString=Group Id: RTICAN1\n  SourceProductName=dSPACE RTI CAN Blockset
  VDC2_0B : Outport
  wires:
  VDC2_0B1/6 -> Bus Creator3/6  "SPN1810_LongitudinalAcceleration"
  VDC2_0B1/5 -> Bus Creator3/5  "LateralAcceleration"
  VDC2_0B1/4 -> Bus Creator3/4  "YawRate"
  VDC2_0B1/3 -> Bus Creator3/3  "SteerWheelAngleSensorType"
  VDC2_0B1/2 -> Bus Creator3/2  "SteerWheelTurnCounter"
  VDC2_0B1/1 -> Bus Creator3/1  "SteerWheelAngle"
  Data Type Conversion9/1 -> Bus Creator3/8  "RX_time"
  Data Type Conversion10/1 -> Bus Creator3/9  "RX_delta_time"
  Data Type Conversion8/1 -> Bus Creator3/7  "RX_status"
  VDC2_0B1/7 -> Data Type Conversion8/1
  VDC2_0B1/8 -> Data Type Conversion9/1
  VDC2_0B1/9 -> Data Type Conversion10/1
  Enable/1 -> VDC2_0B1/Enable
  Bus Creator3/1 -> VDC2_0B/1  "VDC2_0B"

== system SUB_ECU_L4_MABX_HW_Interface_PIC_PB/CAN_PIC_PB/CAN_RX_VEP1_03/RX_CAN_1 ==
  Enable : Inport
  Bus Creator3 : BusCreator  Inputs=8
  Data Type Conversion{1..5,9..10} (7 alike) : DataTypeConversion  OutDataTypeStr=double  SaturateOnIntegerOverflow=on
  Data Type Conversion8 : DataTypeConversion  OutDataTypeStr=boolean  SaturateOnIntegerOverflow=on
  VEP1 : rtican/RTICAN Receive (RX)   Reserved1=[]  Reserved2=[]  Reserved3=[]  Reserved4=[]  SfcnMessage=[]  Msg_Struct=[]  BoardTypeNo=[]  BoardNo=[]  ChannelNo=[]  Parameters=[]  DialogFcn=[]  UnitName=[]  Revision=[]  UnitValues=[]  DSProperties=struct('RTI',struct('Version',uint32(5),'BlockType',struct('isSLSource',uint8(1),'isSLSink',uint8(1),'isHWSource',uint8(0),'isHWSink',uint8(0),'isSetup',uint8(0),'isInline',uint8(1),'isNonInline',uint8(0),'isInterrupt',uint8(0),'isChannelwise',uint8(0)),'IOBoardType','RTICAN','UnitType','MESSAGE','Identifier','RX','DialogType','MSVC','BlockSet','RTICAN','SlaveProcessor','CAN'))  RTIBlockInterface=struct('OutputPortsWidth',int32([1 1 1 1 1 1 1 1]),'OutputPortsActive',[1 1 1 1 1 1 1 1],'OutputPortsName',{{'NetBatteryCurrent','AltCurrent','ChargingSystemPotential','BatteryPotential_PowerInput1','KeyswitchBatteryPotential',['RX status'],['RX time'],['RX delta time']}},'OutputPortsDataType',{{'SS_DOUBLE','SS_DOUBLE','SS_DOUBLE','SS_DOUBLE','SS_DOUBLE','SS_DOUBLE','SS_DOUBLE','SS_DOUBLE'}},'OutputPortsLabel',{{'NetBatteryCurrent','AltCurrent','ChargingSystemPotential','BatteryPotential_PowerInput1','KeyswitchBatteryPotential','','',''}},'OutputPortsLabelMode','ON','InputPortsWidth',int32(0),'InputPortsActive',0,'DialogFcn','rtican_message_interface_gui','BlockDisplay',{{'','center'}},'IconTransparency','on','ParameterTunableNames',{{}},'InitLevel',3,'BlockName',struct('Token',{{'VEP1'}}),'SampleTime',{{-1}},'TriggerPort',{{'none'}},'EnablePort',{{'yes'}})  RTIBlockParameters=struct('BoardTypeNo',{{1,'OFF',[]}},'BoardNo',{{1,'ON',[1 16]}},'ChannelNo',{{1,'ON',[1 2]}},'Parameters',{{struct('DataFileSupport',struct('DataFileSelectedMaster',1,'DataFileSelectedLocal',0,'DataFileName',['c:\users\gavin.coelho\repos\l4 svn\branches\gennaro\project_l4\src\projectlibrary\dbc\mabx_can1.dbc|c:\users\gavin.coelho\repos\l4 svn\branches\gennaro\project_l4\src\projectlibrary\dbc\j1939_famosdbcwithfusion.dbc|'],'DataFileDate',{{{['09-Feb-2018 08:37:30']},{['07-Feb-2018 15:04:58']}}},'SelectedFile',['<no file selected>']),'Options',struct('StatusSelected',1,'TimeSelected',1,'DeltaTimeSelected',1,'BytePortSelected',0,'MessageLengthSelected',0,'TriggerPort',struct('Selected',0,'TriggerType',0),'UserCoding',struct('Selected',0,'InterfaceFile','UserDecodingFile','FcnName','UserDecodeFcn','InportSelected',0,'InportWidth',1,'OutportSelected',0,'OutportWidth',1),'EnablePortSelected',1,'SignalOnPortnameSelected',1,'UseRXService',1),'Message',struct('MsgOnBlocknameSelected',1,'MsgName','VEP1','MsgIdFormat',1,'MsgId',419362563,'MsgLength',8,'NumSignals',5,'SampleTime',-1,'Signal',struct('SgnName',{'NetBatteryCurrent','AltCurrent','ChargingSystemPotential','BatteryPotential_PowerInput1','KeyswitchBatteryPotential'},'SgnStartBit',{0,8,16,32,48},'SgnLength',{8,8,16,16,16},'SgnType',{0,0,0,0,0},'ModeValue',{-1,-1,-1,-1,-1},'DataType',{0,0,0,0,0},'ByteLayout',{0,0,0,0,0},'Factor',{1,1,0.05,0.05,0.05},'Offset',{-125,0,0,0,0},'SgnComment',{{['Net flow of electrical current into/out of the battery or batteries.']},{['Measure of electrical current flow from the alternator.']},{['Electrical potential measured at the charging system output.']},{['This parameter measures the first source of battery potential as measured at the input of the ECM/actuator etc.']},{['Battery potential measured at the input of the electronic control unit supplied through a keyswitch or similar switching']}},'SgnUnit',{'A','A','V','V','V'},'Min',{-125,0,0,0,0},'Max',{125,250,3212.75,3212.75,3212.75},'SLDataType',{'SS_DOUBLE','SS_DOUBLE','SS_DOUBLE','SS_DOUBLE','SS_DOUBLE'}),'MsgIdNumFormat',1,'MsgComment',{{['Vehicle Electrical Power 1']}}),'Version',1.2,'general',struct('isFromLib',0)),'OFF',[]}},'GroupId',{{struct('Group',{{'RTICAN'}},'No',1,'Behavior',{{'NAMECHANGE'}},'BlockType',{{'SINK'}},'NameChangeFlag',0),'OFF',[]}},'SFcnRTICANMessage',{{struct('MsgType','RX','SFcnPortType','Scalar','MsgName','VEP1','MsgIdFormat','XTD','MsgId',419362563,'MsgLength',8,'NumSignals',5,'SampleTime',-1,'Signal',struct('SgnName',{'NetBatteryCurrent','AltCurrent','ChargingSystemPotential','BatteryPotential_PowerInput1','KeyswitchBatteryPotential'},'SgnStartBit',{0,8,16,32,48},'SgnLength',{8,8,16,16,16},'SgnType',{'standard','standard','standard','standard','standard'},'ModeValue',{-1,-1,-1,-1,-1},'DataType',{['unsigned int'],['unsigned int'],['unsigned int'],['unsigned int'],['unsigned int']},'ByteLayout',{['little endian'],['little endian'],['little endian'],['little endian'],['little endian']},'Factor',{1,1,0.05,0.05,0.05},'Offset',{-125,0,0,0,0},'SLDataType',{'SS_DOUBLE','SS_DOUBLE','SS_DOUBLE','SS_DOUBLE','SS_DOUBLE'}),'StatusSelected','yes','TimeSelected','yes','DeltaTimeSelected','yes','BytePortSelected','no','MessageLengthSelected','no','TriggerPort',struct('Selected','no','TriggerType',0),'UserCoding',struct('Selected','no','InterfaceFile','UserDecodingFile','FcnName','UserDecodeFcn','InportSelected','no','InportWidth',1,'OutportSelected','no','OutportWidth',1),'EnablePortSelected','yes','UseRXService','yes','BoardType','DS1','BoardNo',1,'ControllerNo',1),'OFF',[]}},'TLCFileName',{{'rtican_rx_message','OFF',[]}})  RTISFcnParameters=struct('SFcnRTICANMessage','struct','TLCFileName','char')  RTIBlockParaDefault=struct('BoardTypeNo',4302,'BoardNo',1,'ChannelNo',1,'Parameters',struct('DataFileSupport',struct('DataFileSelectedMaster',0,'DataFileSelectedLocal',0,'DataFileName','','DataFileDate','','SelectedFile',['<no file selected>']),'Options',struct('StatusSelected',1,'TimeSelected',1,'DeltaTimeSelected',1,'BytePortSelected',0,'MessageLengthSelected',0,'TriggerPort',struct('Selected',0,'TriggerType','rising'),'UserCoding',struct('Selected',0,'InterfaceFile','UserDecodingFile','FcnName','UserDecodeFcn','InportSelected',0,'InportWidth',1,'OutportSelected',0,'OutportWidth',1),'EnablePortSelected',0,'SignalOnPortnameSelected',1,'UseRXService',0),'Message',struct('MsgOnBlocknameSelected',0,'MsgName',['RX Message'],'MsgIdFormat',0,'MsgId',100,'MsgLength',8,'NumSignals',1,'SampleTime',-1,'Signal',struct('SgnName',['RX signal'],'SgnStartBit',0,'SgnLength',8,'SgnType',0,'ModeValue',-1,'DataType',0,'SLDataType','SS_DOUBLE','ByteLayout',0,'Factor',1,'Offset',0,'Min',0,'Max',255,'SgnComment',{{}},'SgnUnit',''),'MsgIdNumFormat',0,'MsgComment',{{''}}),'Version',1.2,'general',struct('isFromLib',1)),'GroupId',struct('Group',{{'RTICAN'}},'No',1,'Behavior',{{'NAMECHANGE'}},'BlockType',{{'SINK'}},'NameChangeFlag',0),'SFcnRTICANMessage',struct('MsgType','RX','MsgName',['RX Message'],'MsgIdFormat','STD','MsgId',100,'MsgLength',8,'NumSignals',1,'SampleTime',-1,'Signal',struct('SgnName',['RX signal'],'SgnStartBit',0,'SgnLength',8,'SgnType','standard','ModeValue',-1,'DataType',['unsigned int'],'ByteLayout',['little endian'],'SLDataType','SS_DOUBLE','Factor',1,'Offset',0),'StatusSelected','yes','TimeSelected','yes','DeltaTimeSelected','yes','BytePortSelected','no','MessageLengthSelected','no','EnablePortSelected','no','UserCoding',struct('Selected','no','InterfaceFile','UserDecodingFile','FcnName','UserDecodeFcn','InportSelected','no','InportWidth',1,'OutportSelected','no','OutportWidth',1),'TriggerPort',struct('Selected','no','TriggerType','rising'),'UseRXService','no','BoardType','DS4302','BoardNo',1,'ControllerNo',1,'SFcnPortType','Scalar'),'TLCFileName','rtican_rx_message')
      settings: AttributesFormatString=Group Id: RTICAN1\n  SourceProductName=dSPACE RTI CAN Blockset
  VEP1_03 : Outport
  wires:
  Bus Creator3/1 -> VEP1_03/1  "VEP1_03"
  Enable/1 -> VEP1/Enable
  VEP1/8 -> Data Type Conversion10/1
  VEP1/7 -> Data Type Conversion9/1
  VEP1/6 -> Data Type Conversion8/1
  VEP1/2 -> Data Type Conversion2/1  "AltCurrent"
  VEP1/5 -> Data Type Conversion5/1  "KeyswitchBatteryPotential"
  VEP1/4 -> Data Type Conversion4/1  "BatteryPotential_PowerInput1"
  VEP1/3 -> Data Type Conversion3/1  "ChargingSystemPotential"
  VEP1/1 -> Data Type Conversion1/1  "NetBatteryCurrent"
  Data Type Conversion4/1 -> Bus Creator3/4  "BatteryPotential_PowerInput1"
  Data Type Conversion1/1 -> Bus Creator3/1  "PitchAngleExRange"
  Data Type Conversion5/1 -> Bus Creator3/5  "KeyswitchBatteryPotential"
  Data Type Conversion3/1 -> Bus Creator3/3  "ChargingSystemPotential"
  Data Type Conversion2/1 -> Bus Creator3/2  "AltCurrent"
  Data Type Conversion10/1 -> Bus Creator3/8  "RX_delta_time"
  Data Type Conversion9/1 -> Bus Creator3/7  "RX_time"
  Data Type Conversion8/1 -> Bus Creator3/6  "RX_status"

== system SUB_ECU_L4_MABX_HW_Interface_PIC_PB/CAN_PIC_PB/CAN_RX_VI_00/CAN_RX_VI_00 ==
  TPCM : Inport
  TPDT : Inport  Port=2
  timeStamp : Inport  Port=3
  Enable : EnablePort
  Bus Selector1 : BusSelector  OutputSignals=Signals.SPN2572_SequenceNumber
  Bus Selector3 : BusSelector  OutputSignals=Signals.SPN2573_PacketizedData
  Bus Selector4 : BusSelector  OutputSignals=Signals.TPCM_BAM.SPN2568_TotalNumberOfPackets
  Decode : Subsystem  TreatAsAtomicUnit=on
  Demux : Demux  Outputs=7
  Unit Delay : UnitDelay  InitialCondition=uint8(hex2dec('FF')) * ones(17, 1, 'uint8')  SampleTime=-1
  serialize_tpdt : MATLAB Function  TreatAsAtomicUnit=on
  RawData : Outport
  RX_status : Outport  Port=2
  RX_time : Outport  Port=3
  RX_delta_time : Outport  Port=4
  wires:
  timeStamp/1 -> Decode/2(timeStamp)
  Demux/3 -> serialize_tpdt/6(byte3)
  Demux/7 -> serialize_tpdt/10(byte7)
  Demux/6 -> serialize_tpdt/9(byte6)
  Demux/4 -> serialize_tpdt/7(byte4)
  Demux/5 -> serialize_tpdt/8(byte5)
  Demux/2 -> serialize_tpdt/5(byte2)
  Demux/1 -> serialize_tpdt/4(byte1)
  Bus Selector3/1 -> Demux/1  "<SPN2573_PacketizedData>"
  Decode/1(RawData) -> RawData/1  "RawData"
  Decode/3(RX_delta_time) -> RX_delta_time/1  "RX_delta_time"
  Decode/2(RX_time) -> RX_time/1  "RX_time"
  serialize_tpdt/1(RX_status) -> Decode/Enable, RX_status/1  "RX_status"
  serialize_tpdt/2(Data) -> Decode/1(Inport), Unit Delay/1
  Unit Delay/1 -> serialize_tpdt/1(data_packet_previous)
  Bus Selector4/1 -> serialize_tpdt/2(TotalNumberOfPackets)  "<SPN2568_TotalNumberOfPackets>"
  Bus Selector1/1 -> serialize_tpdt/3(SequenceNumber)  "<SPN2572_SequenceNumber>"
  [TPDT] -> Bus Selector3/1, Bus Selector1/1
  [TPCM] -> Bus Selector4/1
  TPDT/1 -> [TPDT]
  TPCM/1 -> [TPCM]
